simulink model "bloques6"  (R2020a)
settings: Solver=VariableStepAuto  StartTime=0.0  StopTime=100  RelTol=1e-3
settings Model: Creator=sht  LastModifiedBy=sht

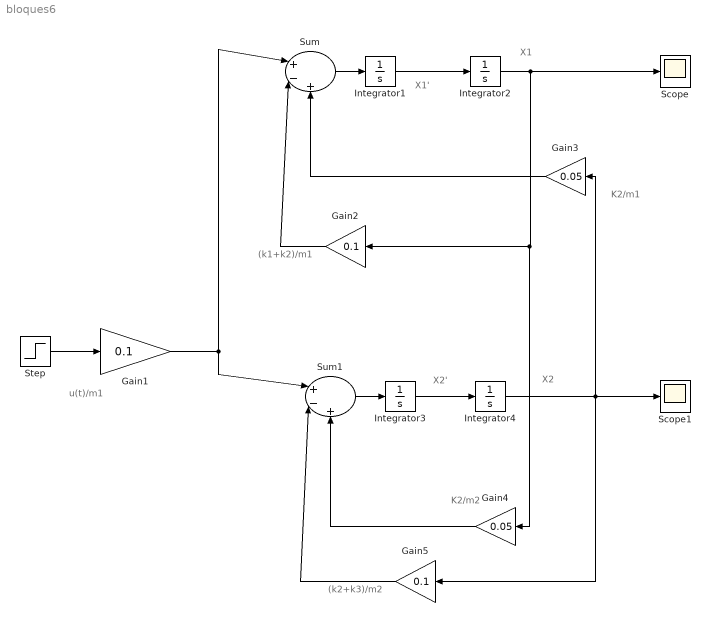
== system bloques6 ==
  note: u(t)/m1
  note: (k1+k2)/m1
  note: (k2+k3)/m2
  note: X2'
  note: X2
  note: X1'
  note: X1
  note: K2/m1
  note: K2/m2
  Gain1 : Gain  Gain=0.1
  Gain2 : Gain  Gain=0.1
  Gain3 : Gain  Gain=0.05
  Gain4 : Gain  Gain=0.05
  Gain5 : Gain  Gain=0.1
  Integrator{1..4} (4 alike) : Integrator  ContinuousStateAttributes='X2'
  Scope : Scope
  Scope1 : Scope
  Step : Step  After=100  SampleTime=0
  Sum : Sum  Inputs=|+-+
  Sum1 : Sum  Inputs=|+-+
  wires:
  Integrator1/1 -> Integrator2/1
  Step/1 -> Gain1/1
  Gain1/1 -> Sum1/1, Sum/1
  Gain2/1 -> Sum/2
  Sum/1 -> Integrator1/1
  Integrator2/1 -> Scope/1, Gain4/1, Gain2/1
  Gain3/1 -> Sum/3
  Gain4/1 -> Sum1/3
  Integrator3/1 -> Integrator4/1
  Sum1/1 -> Integrator3/1
  Integrator4/1 -> Gain5/1, Scope1/1, Gain3/1
  Gain5/1 -> Sum1/2
